simulink model "BlueROV2_Heavy_6DOF"  (R2024a)
settings: Solver=VariableStepAuto  StartTime=0.0  StopTime=100  RelTol=1e-3
values from neighbouring files (symbols this model uses):
  initial_state = zeros(12, 1)    [init_blueROV2Heavy.m]
settings Model: Creator=19486  LastModifiedBy=19486

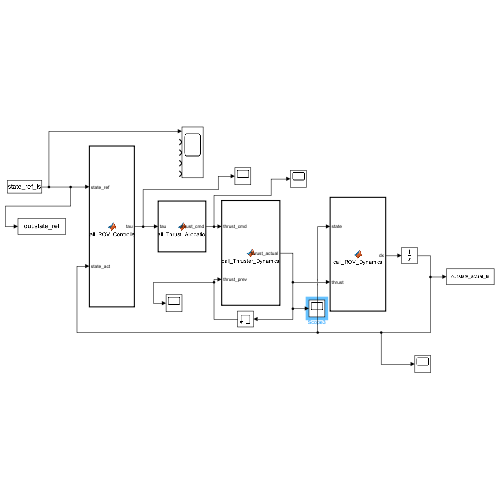
[thumbnail: Simulink's stored preview of the top-level diagram]
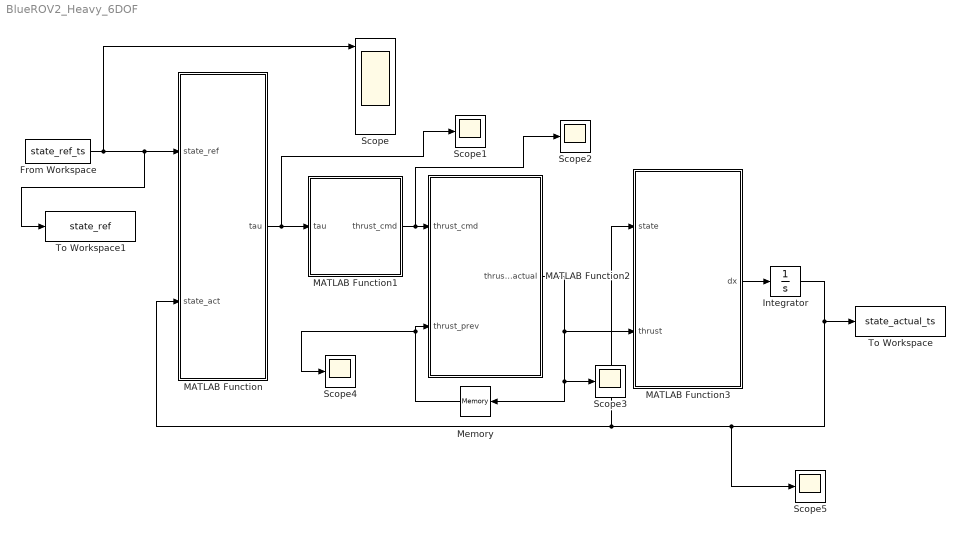
== system BlueROV2_Heavy_6DOF ==
  From Workspace : FromWorkspace  VariableName=state_ref_ts  SampleTime=0.01
  Integrator : Integrator  InitialCondition=initial_state
  MATLAB Function : MATLAB Function  TreatAsAtomicUnit=on
  MATLAB Function1 : MATLAB Function  TreatAsAtomicUnit=on
  MATLAB Function2 : MATLAB Function  TreatAsAtomicUnit=on
  MATLAB Function3 : MATLAB Function  TreatAsAtomicUnit=on
  Memory : Memory
  Scope : Scope  NumInputPorts=5
  Scope{1..5} (5 alike) : Scope
  To Workspace : ToWorkspace  VariableName=state_actual_ts  SaveFormat=Timeseries  SampleTime=0.01
  To Workspace1 : ToWorkspace  VariableName=state_ref  SaveFormat=Timeseries  SampleTime=0.01
  wires:
  From Workspace/1 -> Scope/1, To Workspace1/1, MATLAB Function/1(state_ref)
  MATLAB Function/1(tau) -> Scope1/1, MATLAB Function1/1(tau)
  MATLAB Function2/1(thrust_actual) -> Scope3/1, Memory/1, MATLAB Function3/2(thrust)
  Memory/1 -> Scope4/1, MATLAB Function2/2(thrust_prev)
  MATLAB Function3/1(dx) -> Integrator/1
  Integrator/1 -> Scope5/1, MATLAB Function3/1(state), MATLAB Function/2(state_act), To Workspace/1
  MATLAB Function1/1(thrust_cmd) -> Scope2/1, MATLAB Function2/1(thrust_cmd)

== matlab function BlueROV2_Heavy_6DOF/MATLAB Function1 ==
  settings: updateMethod=DISCRETE  sampleTime=0.01
  data: tau input; thrust_cmd output; params parameter
function thrust_cmd = call_Thrust_Allocation(tau, params)
    thrust_cmd = thrust_alloc(tau, params);
end

== matlab function BlueROV2_Heavy_6DOF/MATLAB Function ==
  settings: updateMethod=DISCRETE  sampleTime=0.01
  data: state_ref input; tau output; state_act input; params parameter
function tau = call_ROV_Controller(state_ref, state_act,params)
    tau = controller_smc2(state_ref, state_act, params);
end

== matlab function BlueROV2_Heavy_6DOF/MATLAB Function2 ==
  settings: updateMethod=DISCRETE  sampleTime=0.01
  data: thrust_cmd input; thrust_actual output; thrust_prev input; params parameter
function thrust_actual = call_Thruster_Dynamics(thrust_cmd, thrust_prev, params)
   thrust_actual = motor_dynamics(thrust_cmd, thrust_prev, params);
end

== matlab function BlueROV2_Heavy_6DOF/MATLAB Function3 ==
  settings: updateMethod=DISCRETE  sampleTime=0.01
  data: state input; dx output size=[12 1]; thrust input; params parameter
function dx = call_ROV_Dynamics(state, thrust, params)
   dx = rov_plant(state, thrust, params);
end
